simulink model "Fig242"  (R2014b)
settings: Solver=ode3  StartTime=0.0  StopTime=10.011  FixedStep=2e-5  RelTol=1e-5
libraries: commutil2 x2, commfilt2 x1, commchan3 x1, commsink2 x1, commrandsrc2 x1
settings Model: Creator=Dennis Silage  LastModifiedBy=Silage
settings DataIOCC: SignalLoggingSaveFormat=ModelDataLogs
settings OptimizationCC: ExpressionDepthLimit=2147483647  InitFltsAndDblsToZero=on
settings DebuggingCC: UnderspecifiedInitializationDetection=Classic  MergeDetectMultiDrivingBlocksExec=none  SolverPrmCheckMsg=none  FcnCallInpInsideContextMsg=UseLocalSettings  StateNameClashWarn=warning
settings GRTTargetCC: CombineOutputUpdateFcns=off  GRTInterface=on

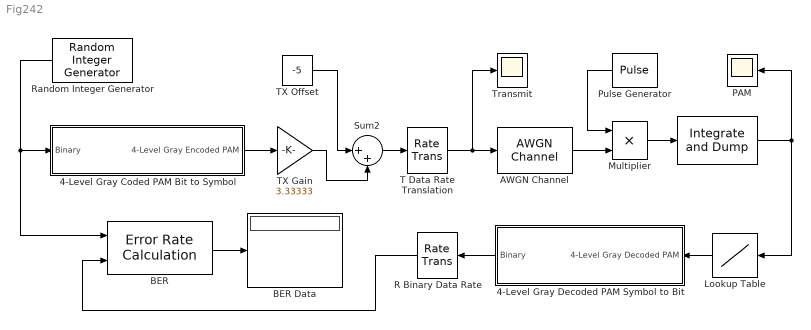
== system Fig242 ==
  " " : commfilt2/Integrate and Dump  obssamples=100  offsetsamples=0  nodump=off  roundingMode=Floor  overflowMode=off
  4-Level Gray Coded PAM Bit to Symbol : Subsystem
  4-Level Gray Decoded PAM Symbol to Bit : Subsystem
  AWGN Channel : commchan3/AWGN Channel  InputProcessing=Inherited (this choice will be removed - see release notes)  seed=randseed  noiseMode="Signal to noise ratio  (Eb/No)"  EbNodB=40  EsNodB=20  SNRdB=10  bitsPerSym=2  Ps=13.89  Tsym=2e-3  variance=0
  BER : commsink2/Error Rate Calculation  N=8  st_delay=4  cp_mode=Entire frame  subframe=[]  PMode=Port  WsName=ErrorVec  RsMode2=off  stop=off  numErr=100  maxBits=1e6
  BER Data : Display
  Lookup Table : Lookup_n-D  NumberOfTableDimensions=1  BreakpointsForDimension1=[-2500, -833.333, 833.333, 2500]  BreakpointsForDimension3=[5, 7]  Table=[0, 1, 2, 3]  InterpMethod=Nearest  InternalRulePriority=Speed  RndMeth=Simplest  InputSameDT=on
  Multiplier : Product  RndMeth=Zero
  PAM : Scope
      settings: TimeRange=0.05  YMin=-8  YMax=8
  Pulse Generator : DiscretePulseGenerator  Amplitude=5  Period=100  PulseWidth=99  SampleTime=2e-5
  "R Binary Data Rate  " : RateTransition  OutPortSampleTime=1e-3
  Random Integer Generator : commrandsrc2/Random Integer Generator  mul=2  seed=randseed  Ts=1e-3  frameBased=off  sampPerFrame=1  orient=off  outDataType=double
  Sum2 : Sum  Inputs=|++
  T Data Rate Translation : RateTransition  OutPortSampleTime=2e-5
  TX Gain : Gain  Gain=3.33333
  TX Offset : Constant  Value=-5
  Transmit : Scope
      settings: TimeRange=0.05  YMin=-8  YMax=8
  wires:
  BER/1 -> BER Data/1
  Multiplier/1 -> " "/1
  AWGN Channel/1 -> Multiplier/2
  Pulse Generator/1 -> Multiplier/1
  T Data Rate Translation/1 -> AWGN Channel/1, Transmit/1
  Random Integer Generator/1 -> 4-Level Gray Coded PAM Bit to Symbol/1(Binary), BER/1
  "R Binary Data Rate  "/1 -> BER/2
  TX Gain/1 -> Sum2/2
  Sum2/1 -> T Data Rate Translation/1
  TX Offset/1 -> Sum2/1
  4-Level Gray Decoded PAM Symbol to Bit/1(Binary) -> "R Binary Data Rate  "/1
  4-Level Gray Coded PAM Bit to Symbol/1("4-Level Gray Encoded PAM ") -> TX Gain/1
  " "/1 -> Lookup Table/1, PAM/1
  Lookup Table/1 -> 4-Level Gray Decoded PAM Symbol to Bit/1(4-Level Gray Decoded PAM)

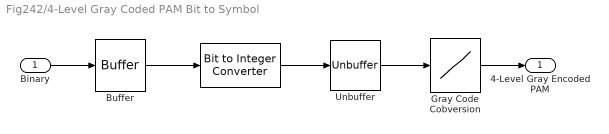
== system Fig242/4-Level Gray Coded PAM Bit to Symbol ==
  Binary : Inport
  " " : commutil2/Bit to Integer Converter  nbits=2  bitOrder=MSB first  signedOutputValues=Unsigned  outDtype=Inherit via internal rule  outDtypeSigned=Inherit via internal rule
  Buffer : Buffer  N=2  TreatMby1Signals=One channel
  "Gray Code Cobversion " : Lookup_n-D  NumberOfTableDimensions=1  BreakpointsForDimension1=[0, 1, 2, 3]  BreakpointsForDimension3=[5, 7]  Table=[0, 1, 3, 2]  InternalRulePriority=Speed  RndMeth=Simplest  InputSameDT=on
  Unbuffer : Unbuffer  SampleBasedProcessing=Same as frame based
  "4-Level Gray Encoded PAM " : Outport
  wires:
  Binary/1 -> Buffer/1
  Buffer/1 -> " "/1
  " "/1 -> Unbuffer/1
  Unbuffer/1 -> "Gray Code Cobversion "/1
  "Gray Code Cobversion "/1 -> "4-Level Gray Encoded PAM "/1

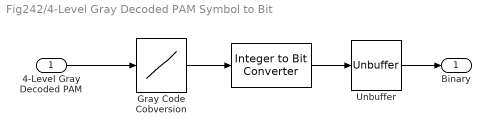
== system Fig242/4-Level Gray Decoded PAM Symbol to Bit ==
  4-Level Gray Decoded PAM : Inport
  " " : commutil2/Integer to Bit Converter  nbits=2  signedInputValues=Unsigned  bitOrder=MSB first  outDtype=Inherit via internal rule
  "Gray Code Cobversion " : Lookup_n-D  NumberOfTableDimensions=1  BreakpointsForDimension1=[0, 1, 2, 3]  BreakpointsForDimension3=[5, 7]  Table=[0, 1, 3, 2]  InternalRulePriority=Speed  RndMeth=Simplest  InputSameDT=on
  Unbuffer : Unbuffer  SampleBasedProcessing=Same as frame based
  Binary : Outport
  wires:
  " "/1 -> Unbuffer/1
  Unbuffer/1 -> Binary/1
  "Gray Code Cobversion "/1 -> " "/1
  4-Level Gray Decoded PAM/1 -> "Gray Code Cobversion "/1
